simulink model "QCar2_Physical_02"  (R2024a)
settings: Solver=ode1  StartTime=0.0  StopTime=inf  FixedStep=Controller_Sample_Time  RelTol=1e-3  EnableMultiTasking=on
PreLoadFcn:
  | QCarSetup
values from neighbouring files (symbols this model uses):
  Audio_Sample_Time = 0.3    [QCarSetup.m]
  CSI_Sample_Time = 1/60    (= 0.0166666666667)    [QCarSetup.m]
  ImageDisplay_Sample_Time = 120*Controller_Sample_Time    (= 0.1)    [QCarSetup.m]
  LiDAR_Sample_Time = CSI_Sample_Time*3    (= 0.05)    [QCarSetup.m]
  NN_Sample_Time = RealSense_Sample_Time*1    (= 0.0333333333333)    [QCarSetup.m]
  RealSense_Sample_Time = CSI_Sample_Time*2    (= 0.0333333333333)    [QCarSetup.m]
undefined symbols (not defined in the file or in its folder): Cobra_Start, DiscIntNeverNeededParam, engine, gcbh, height, HIL, honk, Joystick_Sample_Time, JPEG, left, Point, put_me_down, qc_get_step_size, top, truck_start, video_display_show, width
libraries: quarc_library x53, simulink x4, simulink_extras x1, visiontextngfix x1
(part 1 of 2)
settings Model: SimulationMode=external  ExtModeTrigDuration=10000  Creator=PKaram  LastModifiedBy=admin
settings SolverCC: AlgebraicLoopSolver=TrustRegion  PositivePriorityOrder=on  AutoInsertRateTranBlk=on
settings DataIOCC: ReturnWorkspaceOutputs=off
settings OptimizationCC: ReuseModelBlockBuffer=off
settings DebuggingCC: ParameterPrecisionLossMsg=none  UnconnectedInputMsg=warning  UnconnectedOutputMsg=warning  UnconnectedLineMsg=warning  ArithmeticOperatorsInVariantConditions=warning
settings HardwareCC: ProdBitPerLong=64  ProdLargestAtomicInteger=LongLong  ProdLargestAtomicFloat=Double  ProdLongLongMode=on  ProdHWDeviceType=ARM Compatible->ARM 64-bit (LP64)
settings ModelReferenceCC: EnableRefExpFcnMdlSchedulingChecks=on
settings SFSimCC: SimUseLocalCustomCode=off  CustomCodeUndefinedFunction=UseInterfaceOnly
settings RTWCC: Description=QUARC Linux QCar2 Target Using Toolchain  SystemTargetFile=quarc_linux_qcar2.tlc  TemplateMakefile=quarc_linux_nvidia_tmf  RTWUseLocalCustomCode=off  Toolchain=QUARC linux_qcar2 | gmake (64-bit Windows)  BuildConfiguration=Faster Runs  GPUComputeCapability=3.5  DLArmComputeVersion=19.05
settings CodeAppCC: StateflowObjectComments=on
settings STFCustomTargetCC: ConcurrentExecutionCompliant=on  SystemTargetFile=quarc_linux_qcar2.tlc
settings GRTTargetCC: ParMdlRefBuildCompliant=off  CompOptLevelCompliant=off  CombineOutputUpdateFcns=off  MatFileLogging=off  CPPClassGenCompliant=off  GRTInterface=on  ExtMode=on  ExtModeMexFile=quarc_comm  ExtModeMexArgs='-w -d /tmp -uri %u', 'tcpip://192.168.2.11:17001'
settings ConfigComp: CovMetricSettings=dswe

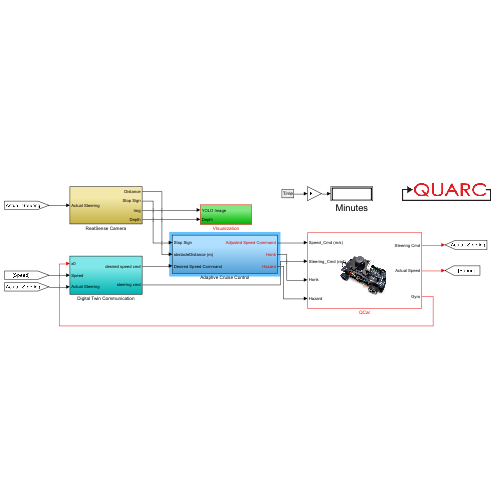
[thumbnail: Simulink's stored preview of the top-level diagram]
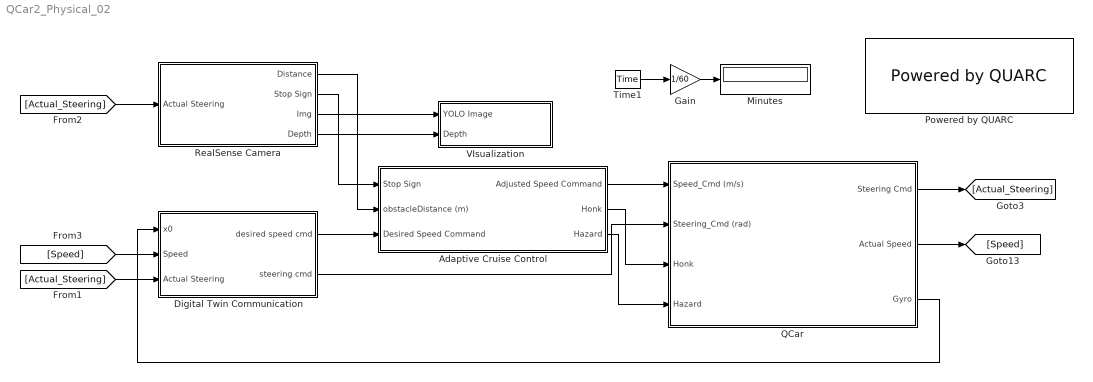
== system QCar2_Physical_02 ==
  Adaptive Cruise Control : Subsystem
  Digital Twin Communication : Subsystem
  Gain : Gain  Gain=1/60
  Minutes : Display
  Powered by QUARC : quarc_library/Logos/Powered by QUARC
  QCar : Subsystem
      mask Display: image('QCar.png'); % Use "Edit Image" on toolstrip to change.
  RealSense Camera : Subsystem
  Time1 : quarc_library/Sources/Time/Time  time_source=Wall clock  sample_time=qc_get_step_size
  VIsualization : Subsystem
  wires:
  QCar/1(Steering Cmd) -> [Actual_Steering]
  Time1/1 -> Gain/1
  Gain/1 -> Minutes/1
  RealSense Camera/1(Distance) -> Adaptive Cruise Control/2(obstacleDistance (m))
  Adaptive Cruise Control/1(Adjusted Speed Command) -> QCar/1(Speed_Cmd (m/s))
  Adaptive Cruise Control/2(Honk) -> QCar/3(Honk)
  QCar/2(Actual Speed) -> [Speed]
  [Actual_Steering] -> RealSense Camera/1(Actual Steering)
  RealSense Camera/2(Stop Sign) -> Adaptive Cruise Control/1(Stop Sign)
  Adaptive Cruise Control/3(Hazard) -> QCar/4(Hazard)
  QCar/3(Gyro) -> Digital Twin Communication/1(x0)
  [Speed] -> Digital Twin Communication/2(Speed)
  [Actual_Steering] -> Digital Twin Communication/3(Actual Steering)
  Digital Twin Communication/2(steering cmd) -> QCar/2(Steering_Cmd (rad))
  Digital Twin Communication/1(desired speed cmd) -> Adaptive Cruise Control/3(Desired Speed Command)
  RealSense Camera/3(Img) -> VIsualization/1(YOLO Image)
  RealSense Camera/4(Depth) -> VIsualization/2(Depth)

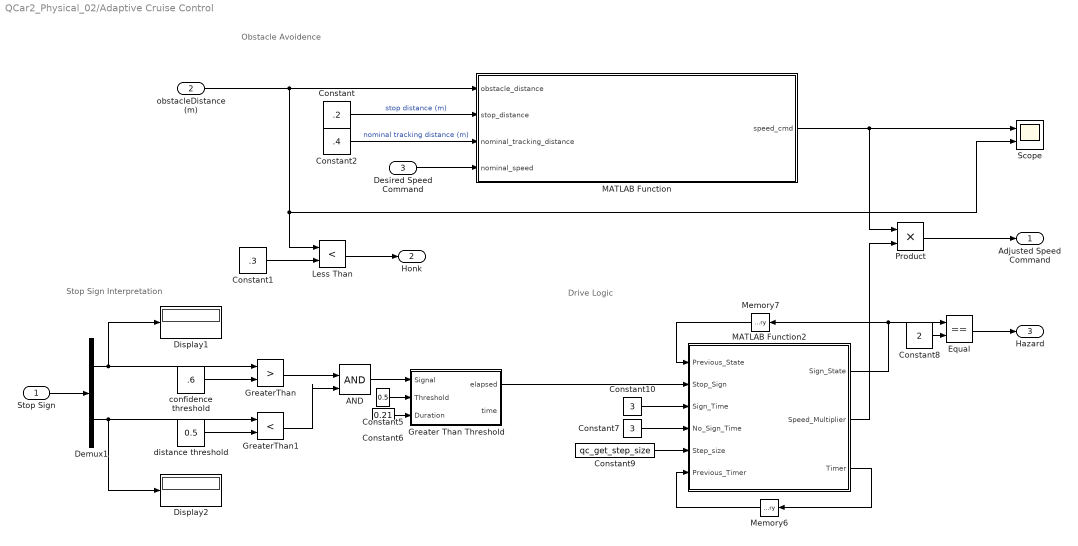
== system QCar2_Physical_02/Adaptive Cruise Control ==
  note: Drive Logic
  note: Obstacle Avoidence
  note: Stop Sign Interpretation
  Stop Sign : Inport
  obstacleDistance (m) : Inport  Port=2
  Desired Speed Command : Inport  Port=3
  AND : Logic  IconShape=distinctive  AllPortsSameDT=off
  Constant : Constant  Value=.2
  Constant1 : Constant  Value=.3
  Constant10 : Constant  Value=3
  Constant2 : Constant  Value=.4
  Constant5 : Constant  Value=0.5
  Constant6 : Constant  Value=0.21
  Constant7 : Constant  Value=3
  Constant8 : Constant  Value=2
  Constant9 : Constant  Value=qc_get_step_size
  Demux1 : Demux  Outputs=2
  Display1 : Display
  Display2 : Display
  Equal : RelationalOperator  Operator===  OutDataTypeStr=boolean  RndMeth=Simplest  InputSameDT=off
  Greater Than Threshold : Subsystem
  GreaterThan : RelationalOperator  Operator=>  OutDataTypeStr=boolean  RndMeth=Simplest  InputSameDT=off
  GreaterThan1 : RelationalOperator  Operator=<  OutDataTypeStr=boolean  RndMeth=Simplest  InputSameDT=off
  Less Than : RelationalOperator  Operator=<  OutDataTypeStr=boolean  RndMeth=Simplest  InputSameDT=off
  MATLAB Function : MATLAB Function  TreatAsAtomicUnit=on
  MATLAB Function2 : MATLAB Function  TreatAsAtomicUnit=on
  Memory6 : Memory  InheritSampleTime=on  LinearizeMemory=on  LinearizeAsDelay=on
  Memory7 : Memory  InitialCondition=1  InheritSampleTime=on  LinearizeMemory=on  LinearizeAsDelay=on
  Product : Product
  Scope : Scope  NumInputPorts=2
  confidence threshold : Constant  Value=.6
  distance threshold : Constant  Value=0.5
  Adjusted Speed Command : Outport  VectorParamsAs1DForOutWhenUnconnected=off
  Honk : Outport  Port=2
  Hazard : Outport  Port=3
  wires:
  Constant2/1 -> MATLAB Function/3(nominal_tracking_distance)  "nominal tracking distance (m)"
  Constant/1 -> MATLAB Function/2(stop_distance)  "stop distance (m)"
  obstacleDistance (m)/1 -> Less Than/1, Scope/2, MATLAB Function/1(obstacle_distance)
  Constant1/1 -> Less Than/2
  Less Than/1 -> Honk/1
  MATLAB Function/1(speed_cmd) -> Scope/1, Product/1
  Desired Speed Command/1 -> MATLAB Function/4(nominal_speed)
  Memory7/1 -> MATLAB Function2/1(Previous_State)
  Memory6/1 -> MATLAB Function2/6(Previous_Timer)
  MATLAB Function2/1(Sign_State) -> Equal/1, Memory7/1
  Constant9/1 -> MATLAB Function2/5(Step_size)
  Constant7/1 -> MATLAB Function2/4(No_Sign_Time)
  MATLAB Function2/2(Speed_Multiplier) -> Product/2
  Constant10/1 -> MATLAB Function2/3(Sign_Time)
  MATLAB Function2/3(Timer) -> Memory6/1
  Product/1 -> Adjusted Speed Command/1
  Stop Sign/1 -> Demux1/1
  Demux1/1 -> GreaterThan/1, Display1/1
  Demux1/2 -> Display2/1, GreaterThan1/1
  confidence threshold/1 -> GreaterThan/2
  distance threshold/1 -> GreaterThan1/2
  GreaterThan/1 -> AND/1
  GreaterThan1/1 -> AND/2
  AND/1 -> Greater Than Threshold/1(Signal)
  Constant5/1 -> Greater Than Threshold/2(Threshold)
  Constant6/1 -> Greater Than Threshold/3(Duration)
  Greater Than Threshold/1(elapsed) -> MATLAB Function2/2(Stop_Sign)
  Equal/1 -> Hazard/1
  Constant8/1 -> Equal/2

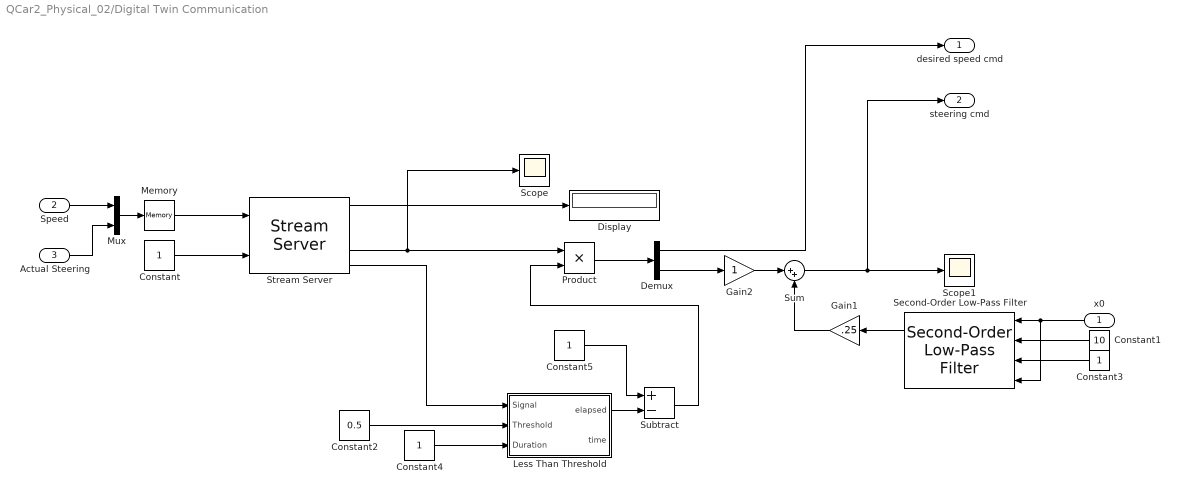
== system QCar2_Physical_02/Digital Twin Communication ==
  x0 : Inport
  Speed : Inport  Port=2
  Actual Steering : Inport  Port=3
  Constant{,3..5} (4 alike) : Constant
  Constant1 : Constant  Value=10
  Constant2 : Constant  Value=0.5
  Demux : Demux  Outputs=2
  Display : Display
  Gain1 : Gain  Gain=.25
  Gain2 : Gain
  Less Than Threshold : Subsystem
  Memory : Memory  InitialCondition=[0 0]
  Mux : Mux  Inputs=2
  Product : Product
  Scope : Scope
  Scope1 : Scope
  Second-Order Low-Pass Filter : quarc_library/Continuous/Second-Order Low-Pass Filter  params_source=External (input ports)  input_width=10  input_zeta=1  input_init=0
  Stream Server : quarc_library/Communications/Basic/Stream Server  uri_source=Specify via dialog (do not evaluate)  uri=tcpip://localhost:777  send_buffer_size=1460  receive_buffer_size=1460  byte_order=little endian (Intel - LSB first)  optimization=Minimum latency  send_options=Send most recent data  receive_options=Receive most recent data  default_value=[0 0]  sample_time=qc_get_step_size  active=off  implementation=Use blocking I/O in a separate thread  send_fifo_size=1000  receive_fifo_size=1000  send_priority=0  receive_priority=0  send_dimensions=off  receive_dimensions=off  max_dimensions=-1  data_type=Inherited via back propagation  type_expr=BusObject
      settings: AttributesFormatString="\"tcpip://localhost:777\""
  Subtract : Sum  Inputs=+-
  Sum : Sum  Inputs=|++
  desired speed cmd : Outport
  steering cmd : Outport  Port=2
  wires:
  Sum/1 -> steering cmd/1, Scope1/1
  Speed/1 -> Mux/1
  Constant1/1 -> Second-Order Low-Pass Filter/2
  Stream Server/1 -> Display/1
  x0/1 -> Second-Order Low-Pass Filter/4, Second-Order Low-Pass Filter/1
  Memory/1 -> Stream Server/1
  Demux/2 -> Gain2/1
  Gain1/1 -> Sum/2
  Less Than Threshold/1(elapsed) -> Subtract/2
  Constant2/1 -> Less Than Threshold/2(Threshold)
  Constant4/1 -> Less Than Threshold/3(Duration)
  Subtract/1 -> Product/2
  Stream Server/4 -> Scope/1, Product/1
  Actual Steering/1 -> Mux/2
  Constant3/1 -> Second-Order Low-Pass Filter/3
  Second-Order Low-Pass Filter/1 -> Gain1/1
  Mux/1 -> Memory/1
  Gain2/1 -> Sum/1
  Stream Server/5 -> Less Than Threshold/1(Signal)
  Constant5/1 -> Subtract/1
  Constant/1 -> Stream Server/2
  Product/1 -> Demux/1
  Demux/1 -> desired speed cmd/1

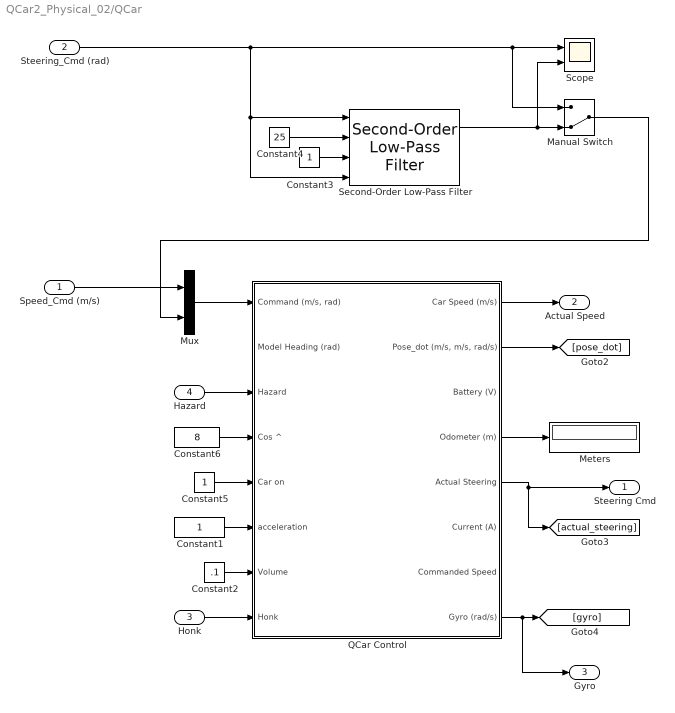
== system QCar2_Physical_02/QCar ==
  Speed_Cmd (m/s) : Inport
  Steering_Cmd (rad) : Inport  Port=2
  Honk : Inport  Port=3
  Hazard : Inport  Port=4
  Constant1 : Constant
  Constant2 : Constant  Value=.1
  Constant3 : Constant
  Constant4 : Constant  Value=25
  Constant5 : Constant
  Constant6 : Constant  Value=8
  Manual Switch : ManualSwitch  CurrentSetting=0
  Meters : Display
  Mux : Mux  Inputs=2
  QCar Control : Subsystem
  Scope : Scope  NumInputPorts=2
  Second-Order Low-Pass Filter : quarc_library/Continuous/Second-Order Low-Pass Filter  params_source=External (input ports)  input_width=1  input_zeta=1  input_init=0
  Steering Cmd : Outport
  Actual Speed : Outport  Port=2
  Gyro : Outport  Port=3
  wires:
  Mux/1 -> QCar Control/1("Command (m/s, rad)")
  Speed_Cmd (m/s)/1 -> Mux/1
  QCar Control/1(Car Speed (m/s)) -> Actual Speed/1
  QCar Control/2("Pose_dot (m/s, m/s, rad/s)") -> [pose_dot]
  QCar Control/5(Actual Steering) -> [actual_steering], Steering Cmd/1
  Constant6/1 -> QCar Control/4(Cos ^)
  Constant1/1 -> QCar Control/6(acceleration)
  Constant5/1 -> QCar Control/5(Car on)
  Constant2/1 -> QCar Control/7(Volume)
  Honk/1 -> QCar Control/8(Honk)
  QCar Control/4(Odometer (m)) -> Meters/1
  Hazard/1 -> QCar Control/3(Hazard)
  Manual Switch/1 -> Mux/2
  Second-Order Low-Pass Filter/1 -> Scope/2, Manual Switch/2
  Steering_Cmd (rad)/1 -> Manual Switch/1, Scope/1, Second-Order Low-Pass Filter/1, Second-Order Low-Pass Filter/4
  Constant3/1 -> Second-Order Low-Pass Filter/3
  Constant4/1 -> Second-Order Low-Pass Filter/2
  QCar Control/8(Gyro (rad/s)) -> Gyro/1, [gyro]

== system QCar2_Physical_02/RealSense Camera ==
  Actual Steering : Inport
  Constant8 : Constant  Value=50
  Constant9 : Constant
  Distance Comparison : Scope  Commented=on  NumInputPorts=3
  NN Classification : Scope
  Obstacle Detection : Subsystem
  Rate Transition : RateTransition
  Rate Transition2 : RateTransition
  Rate Transition4 : RateTransition
  RealSense Capture : Subsystem
  Second-Order Low-Pass Filter2 : quarc_library/Continuous/Second-Order Low-Pass Filter  params_source=External (input ports)  input_width=1  input_zeta=1  input_init=0
  Selector : Selector  NumberOfDimensions=2  InputPortWidth=3  IndexOptions=Index vector (dialog),Select all  Indices=2,1  OutputSizes=1,1
  Terminator : Terminator
  Transfer Fcn : TransferFcn  Numerator=[10]  Denominator=[1 10]
  Distance : Outport
  Stop Sign : Outport  Port=2
  Img : Outport  Port=3
  Depth : Outport  Port=4
  wires:
  Transfer Fcn/1 -> Rate Transition4/1
  Actual Steering/1 -> Transfer Fcn/1
  Constant9/1 -> Second-Order Low-Pass Filter2/3
  Rate Transition2/1 -> Second-Order Low-Pass Filter2/4, Second-Order Low-Pass Filter2/1
  Second-Order Low-Pass Filter2/2 -> Terminator/1
  RealSense Capture/2(New) -> Obstacle Detection/Enable
  Rate Transition4/1 -> Obstacle Detection/2(steering (rad))
  Constant8/1 -> Second-Order Low-Pass Filter2/2
  Second-Order Low-Pass Filter2/1 -> Distance/1, Distance Comparison/1
  RealSense Capture/4(Depth Aligned) -> Obstacle Detection/1(imageDepth)
  RealSense Capture/1(Classification Info) -> Rate Transition/1
  RealSense Capture/3(yolo image) -> Img/1
  Obstacle Detection/2(imageDepthForDisplay) -> Depth/1
  Selector/1 -> Stop Sign/1
  Rate Transition/1 -> NN Classification/1, Selector/1
  Obstacle Detection/1(distance (m)) -> Rate Transition2/1

== system QCar2_Physical_02/VIsualization ==
  YOLO Image : Inport
  Depth : Inport  Port=2
  Body Frame : quarc_library/Sinks/Figures/Polar Figure  figure_mode=Use figure window  figure_tag=figure1  axes_tag=axes1  plot_mode=Frame-based  minimum_rho=0  maximum_rho=4  minimum_theta=0  maximum_theta=360  zero_location=right  direction=clockwise  buffer_size=SPR  update_rate=1  sample_time=-1  initial_position="-1533.6667     -397.66667      638.66667      278.66667"  initial_visibility=off  line1_style=None  line1_width=0.5  line1_color=[0 0.4470 0.7410]  marker1=Point (.)  marker1_size=5  marker1_edge_color=[0 0.447059 0.741176]  marker1_face_color=[0 0.447059 0.741176]  line2_style=Solid line (-)  line2_width=0.5  line2_color=[0.85098 0.32549 0.0980392]  marker2=None  marker2_size=6  marker2_edge_color=[0.85098 0.32549 0.0980392]  marker2_face_color=[0.85098 0.32549 0.0980392]  line3_style=Solid line (-)  line3_width=0.5  line3_color=[0.929412 0.694118 0.12549]  marker3=None  marker3_size=6  marker3_edge_color=[0.929412 0.694118 0.12549]  marker3_face_color=[0.929412 0.694118 0.12549]  line4_style=Solid line (-)  line4_width=0.5  line4_color=[0.494118 0.184314 0.556863]  marker4=None  marker4_size=6  marker4_edge_color=[0.494118 0.184314 0.556863]  marker4_face_color=[0.494118 0.184314 0.556863]  line5_style=Solid line (-)  line5_width=0.5  line5_color=[0.466667 0.67451 0.188235]  marker5=None  marker5_size=6  marker5_edge_color=[0.466667 0.67451 0.188235]  marker5_face_color=[0.466667 0.67451 0.188235]
      settings: SourceProductName=QUARC Targets
  LiDAR : Subsystem
  Newer Depth : Subsystem  LoadFcn=set_param(gcbh, 'UserData', gcb);  StartFcn=video_display_show([gcb, '/Video Display'], 'add', gcb);  mask(Video Compressed Display){algorithm=JPEG, quality=50, sample_time=-1, use_hardware=on}
      mask prompts: algorithm "Compression algorithm:"; quality "Compression quality (0-100):"; sample_time "Sample time (seconds):"; use_hardware "Use hardware acceleration for video display"
      mask help: Displays a video stream on the host, using compression to minimize bandwidth.
      mask init:
      | qc_set_display('Video\nCompressed\nDisplay');
      settings: UndoDeleteFcn=set_param(gcbh, 'UserData', gcb);  OpenFcn=video_display_show([gcb, '/Video Display'], 'show', gcb);  PreDeleteFcn=video_display_show([gcb, '/Video Display'], 'delete');
      settings: CopyFcn=|
      | set_param(gcbh, 'UserData', gcb);
      | set_param(gcbh, 'LinkStatus', 'none');
      settings: NameChangeFcn=|
      | video_display_show([get_param(gcbh, 'UserData'), '/Video Display'], 'rename', [gcb, '/Video Display']);
      | video_display_show([gcb, '/Video Display'], 'add', gcb);
      | set_param(gcbh, 'UserData', gcb);
      mask Help: web(qc_get_block_help_path(gcb));
      mask TypeOptions algorithm: Image Compress/algorithm
      mask TypeOptions quality: Image Compress/quality
      mask TypeOptions sample_time: Video Display/sample_time
      mask TypeOptions use_hardware: Video Display/use_hardware
      mask Display:
      | patch([0.98591 0.98591 0.62618 0.59072 0.56147   0.536   0.536  0.5441 0.56912 0.59207 0.60881 0.62276 0.63527 0.64364  0.6485  0.6485 0.64706 0.64499 0.63662 0.62411 0.61232 0.59837 0.58307 0.56147   0.536   0.536  0.5441  0.5747 0.60953 0.63662 0.67001  0.7034 0.72851 0.75425 0.77927 0.80294 0.82454 0.84119 0.85865 0.87395 0.88574 0.89339  0.8969 0.89969 0.89969 0.89267  0.8816 0.87044 0.85649  0.8384 0.81824 0.80294 0.78764 0.77513 0.76676 0.75776 0.76397 0.77513 0.79178 0.80987 0.82796 0.84326 0.86207 0.98528],[0.18689 0.05522 0.05522 0.05171 0.05171    0.05 0.18338 0.18338 0.19148 0.20435 0.22298 0.24863 0.28589 0.33125 0.38138 0.55139 0.59801 0.63761 0.68189 0.72149 0.74939 0.76694 0.77855 0.79367 0.79952 0.92768 0.92768 0.92768 0.92417 0.92066 0.91364  0.9032 0.89384 0.88106 0.86594 0.85073 0.82634 0.80537 0.77855 0.74363 0.70403 0.65858 0.61079 0.59099 0.41513 0.37202 0.31847 0.29048 0.25556 0.23342  0.2102 0.19382 0.18221 0.17285 0.16943 0.16124  0.1589 0.16241 0.16709 0.17168  0.1787 0.18221 0.18689 0.18689],[0.9,0.90,0.91])
      | patch([0.536 0.52601 0.46823 0.44528 0.41603 0.39101 0.35555 0.33116 0.31451 0.29291  0.2804 0.26717 0.25322 0.23999 0.22406 0.20732 0.19337 0.17528 0.15935 0.14396 0.13217 0.11759 0.10922 0.10085 0.09671 0.09392 0.09041 0.08906 0.08906 0.09464  0.0995 0.10778 0.11894 0.13145 0.14675 0.16349 0.17672 0.19409 0.20732 0.22406 0.23999 0.26159 0.27833 0.29849 0.31793 0.33602 0.35411 0.37085 0.39245 0.41603   0.536   0.536 0.53159 0.46409   0.446 0.42026 0.39587 0.37571 0.36113 0.34925 0.34088 0.33809 0.33809 0.34088 0.34583 0.35627 0.36392 0.38129 0.39587 0.41117 0.42719 0.44672  0.4676 0.48353 0.48353 0.52394   0.536],[0.05 0.04829 0.04712 0.04712 0.04829 0.05063 0.05405 0.05873 0.06107 0.06692 0.07043 0.07619 0.08087 0.08672 0.09482 0.10652 0.11696 0.13325  0.1508 0.17168 0.19499 0.22415 0.25439 0.28472 0.31379 0.35456 0.38489 0.41513 0.58055 0.63878 0.68774 0.72149 0.75641 0.78089 0.80537 0.82859 0.84029 0.85658 0.86594 0.87404  0.8834 0.89267 0.90086 0.90788 0.91247 0.91832 0.92066   0.923 0.92651 0.92768 0.92768 0.79952 0.79952 0.79952 0.79718 0.78899 0.77153 0.75056 0.72149 0.68072 0.62249  0.5549 0.41396 0.37085 0.33242 0.28121 0.25205 0.22181 0.20552 0.19499 0.18572 0.18221 0.17753 0.17636 0.17753  0.1787  0.1787],[0.9,0.90,0.91])
      | disp('Video\nCompressed\nDisplay');
  Rate Timing Plots : Subsystem
  Speed_Tracking : Scope  NumInputPorts=2
  Yolo Image : Subsystem  LoadFcn=set_param(gcbh, 'UserData', gcb);  StartFcn=video_display_show([gcb, '/Video Display'], 'add', gcb);  mask(Video Compressed Display){algorithm=JPEG, quality=50, sample_time=-1, use_hardware=on}
      mask prompts: algorithm "Compression algorithm:"; quality "Compression quality (0-100):"; sample_time "Sample time (seconds):"; use_hardware "Use hardware acceleration for video display"
      mask help: Displays a video stream on the host, using compression to minimize bandwidth.
      mask init:
      | qc_set_display('Video\nCompressed\nDisplay');
      settings: UndoDeleteFcn=set_param(gcbh, 'UserData', gcb);  OpenFcn=video_display_show([gcb, '/Video Display'], 'show', gcb);  PreDeleteFcn=video_display_show([gcb, '/Video Display'], 'delete');
      settings: CopyFcn=|
      | set_param(gcbh, 'UserData', gcb);
      | set_param(gcbh, 'LinkStatus', 'none');
      settings: NameChangeFcn=|
      | video_display_show([get_param(gcbh, 'UserData'), '/Video Display'], 'rename', [gcb, '/Video Display']);
      | video_display_show([gcb, '/Video Display'], 'add', gcb);
      | set_param(gcbh, 'UserData', gcb);
      mask Help: web(qc_get_block_help_path(gcb));
      mask TypeOptions algorithm: Image Compress/algorithm
      mask TypeOptions quality: Image Compress/quality
      mask TypeOptions sample_time: Video Display/sample_time
      mask TypeOptions use_hardware: Video Display/use_hardware
      mask Display:
      | patch([0.98591 0.98591 0.62618 0.59072 0.56147   0.536   0.536  0.5441 0.56912 0.59207 0.60881 0.62276 0.63527 0.64364  0.6485  0.6485 0.64706 0.64499 0.63662 0.62411 0.61232 0.59837 0.58307 0.56147   0.536   0.536  0.5441  0.5747 0.60953 0.63662 0.67001  0.7034 0.72851 0.75425 0.77927 0.80294 0.82454 0.84119 0.85865 0.87395 0.88574 0.89339  0.8969 0.89969 0.89969 0.89267  0.8816 0.87044 0.85649  0.8384 0.81824 0.80294 0.78764 0.77513 0.76676 0.75776 0.76397 0.77513 0.79178 0.80987 0.82796 0.84326 0.86207 0.98528],[0.18689 0.05522 0.05522 0.05171 0.05171    0.05 0.18338 0.18338 0.19148 0.20435 0.22298 0.24863 0.28589 0.33125 0.38138 0.55139 0.59801 0.63761 0.68189 0.72149 0.74939 0.76694 0.77855 0.79367 0.79952 0.92768 0.92768 0.92768 0.92417 0.92066 0.91364  0.9032 0.89384 0.88106 0.86594 0.85073 0.82634 0.80537 0.77855 0.74363 0.70403 0.65858 0.61079 0.59099 0.41513 0.37202 0.31847 0.29048 0.25556 0.23342  0.2102 0.19382 0.18221 0.17285 0.16943 0.16124  0.1589 0.16241 0.16709 0.17168  0.1787 0.18221 0.18689 0.18689],[0.9,0.90,0.91])
      | patch([0.536 0.52601 0.46823 0.44528 0.41603 0.39101 0.35555 0.33116 0.31451 0.29291  0.2804 0.26717 0.25322 0.23999 0.22406 0.20732 0.19337 0.17528 0.15935 0.14396 0.13217 0.11759 0.10922 0.10085 0.09671 0.09392 0.09041 0.08906 0.08906 0.09464  0.0995 0.10778 0.11894 0.13145 0.14675 0.16349 0.17672 0.19409 0.20732 0.22406 0.23999 0.26159 0.27833 0.29849 0.31793 0.33602 0.35411 0.37085 0.39245 0.41603   0.536   0.536 0.53159 0.46409   0.446 0.42026 0.39587 0.37571 0.36113 0.34925 0.34088 0.33809 0.33809 0.34088 0.34583 0.35627 0.36392 0.38129 0.39587 0.41117 0.42719 0.44672  0.4676 0.48353 0.48353 0.52394   0.536],[0.05 0.04829 0.04712 0.04712 0.04829 0.05063 0.05405 0.05873 0.06107 0.06692 0.07043 0.07619 0.08087 0.08672 0.09482 0.10652 0.11696 0.13325  0.1508 0.17168 0.19499 0.22415 0.25439 0.28472 0.31379 0.35456 0.38489 0.41513 0.58055 0.63878 0.68774 0.72149 0.75641 0.78089 0.80537 0.82859 0.84029 0.85658 0.86594 0.87404  0.8834 0.89267 0.90086 0.90788 0.91247 0.91832 0.92066   0.923 0.92651 0.92768 0.92768 0.79952 0.79952 0.79952 0.79718 0.78899 0.77153 0.75056 0.72149 0.68072 0.62249  0.5549 0.41396 0.37085 0.33242 0.28121 0.25205 0.22181 0.20552 0.19499 0.18572 0.18221 0.17753 0.17636 0.17753  0.1787  0.1787],[0.9,0.90,0.91])
      | disp('Video\nCompressed\nDisplay');
  wires:
  YOLO Image/1 -> Yolo Image/1(In1)
  LiDAR/1(Distance) -> Body Frame/1
  LiDAR/2(Heading) -> Body Frame/2
  Depth/1 -> Newer Depth/1(In1)
  [desiredSpd] -> Speed_Tracking/1
  [measuredSpd] -> Speed_Tracking/2

== system QCar2_Physical_02/Adaptive Cruise Control/Greater Than Threshold ==
  Signal : Inport
  Threshold : Inport  Port=2
  Duration : Inport  Port=3
  Data Type Conversion : DataTypeConversion  SaturateOnIntegerOverflow=off  RndMeth=Floor
  Discrete-Time Integrator : DiscreteIntegrator  Priority=1  ExternalReset=level  SampleTime=qc_get_step_size  ICPrevOutput=DiscIntNeverNeededParam  ICPrevScaledInput=DiscIntNeverNeededParam
  Logical Operator : Logic  Operator=NOT  AllPortsSameDT=off  OutDataTypeStr=boolean
  Relational Operator : RelationalOperator  InputSameDT=off
  Relational Operator1 : RelationalOperator  InputSameDT=off
  elapsed : Outport  VectorParamsAs1DForOutWhenUnconnected=off
  time : Outport  Port=2  VectorParamsAs1DForOutWhenUnconnected=off
  wires:
  Data Type Conversion/1 -> Discrete-Time Integrator/1
  Signal/1 -> Relational Operator/1
  Threshold/1 -> Relational Operator/2
  Relational Operator/1 -> Data Type Conversion/1, Logical Operator/1
  Logical Operator/1 -> Discrete-Time Integrator/2
  Discrete-Time Integrator/1 -> Relational Operator1/1, time/1
  Duration/1 -> Relational Operator1/2
  Relational Operator1/1 -> elapsed/1

== system QCar2_Physical_02/Digital Twin Communication/Less Than Threshold ==
  Signal : Inport
  Threshold : Inport  Port=2
  Duration : Inport  Port=3
  Data Type Conversion : DataTypeConversion  SaturateOnIntegerOverflow=off  RndMeth=Floor
  Discrete-Time Integrator : DiscreteIntegrator  Priority=1  ExternalReset=level  SampleTime=qc_get_step_size  ICPrevOutput=DiscIntNeverNeededParam  ICPrevScaledInput=DiscIntNeverNeededParam
  Logical Operator : Logic  Operator=NOT  AllPortsSameDT=off  OutDataTypeStr=boolean
  Relational Operator : RelationalOperator  Operator=<  InputSameDT=off
  Relational Operator1 : RelationalOperator  InputSameDT=off
  elapsed : Outport  VectorParamsAs1DForOutWhenUnconnected=off
  time : Outport  Port=2  VectorParamsAs1DForOutWhenUnconnected=off
  wires:
  Relational Operator1/1 -> elapsed/1
  Duration/1 -> Relational Operator1/2
  Discrete-Time Integrator/1 -> time/1, Relational Operator1/1
  Logical Operator/1 -> Discrete-Time Integrator/2
  Relational Operator/1 -> Logical Operator/1, Data Type Conversion/1
  Threshold/1 -> Relational Operator/2
  Signal/1 -> Relational Operator/1
  Data Type Conversion/1 -> Discrete-Time Integrator/1

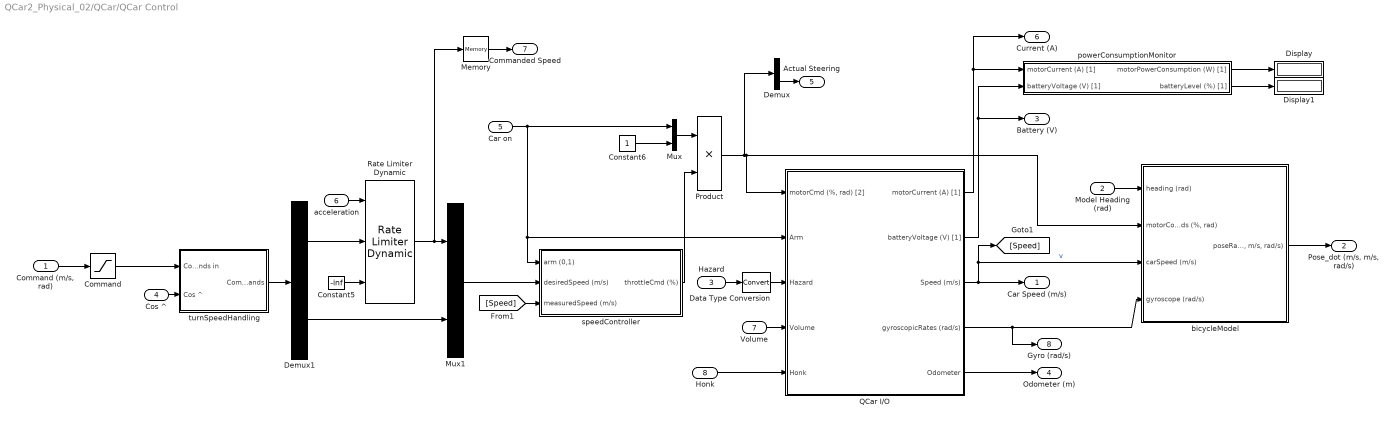
== system QCar2_Physical_02/QCar/QCar Control ==
  "Command (m/s, rad)" : Inport
  Model Heading (rad) : Inport  Port=2
  Hazard : Inport  Port=3
  Cos ^ : Inport  Port=4
  Car on : Inport  Port=5
  acceleration : Inport  Port=6
  Volume : Inport  Port=7
  Honk : Inport  Port=8
  Command : Saturate  UpperLimit=[3 .6]  LowerLimit=-[3 .6]
  Constant5 : Constant  Value=-inf
  Constant6 : Constant
  Data Type Conversion : DataTypeConversion  SaturateOnIntegerOverflow=off  RndMeth=Floor
  Demux : Demux  Outputs=2
  Demux1 : Demux  Outputs=2
  Display : Display
      settings: Decimation=100
  Display1 : Display
      settings: Decimation=100
  Memory : Memory
  Mux : Mux  Inputs=2
  Mux1 : Mux  Inputs=2
  Product : Product
  QCar I/O : Subsystem
  Rate Limiter Dynamic : simulink/Discontinuities/Rate Limiter Dynamic
  bicycleModel : Subsystem
  powerConsumptionMonitor : Subsystem
  speedController : Subsystem
  turnSpeedHandling : Subsystem
  Car Speed (m/s) : Outport
  "Pose_dot (m/s, m/s, rad/s)" : Outport  Port=2
  Battery (V) : Outport  Port=3
  Odometer (m) : Outport  Port=4
  Actual Steering : Outport  Port=5
  Current (A) : Outport  Port=6
  Commanded Speed : Outport  Port=7
  Gyro (rad/s) : Outport  Port=8
  wires:
  QCar I/O/2(batteryVoltage (V) [1]) -> Battery (V)/1, powerConsumptionMonitor/2(batteryVoltage (V) [1])
  powerConsumptionMonitor/1(motorPowerConsumption (W) [1]) -> Display/1
  QCar I/O/1(motorCurrent (A) [1]) -> Current (A)/1, powerConsumptionMonitor/1(motorCurrent (A) [1])
  Model Heading (rad)/1 -> bicycleModel/1(heading (rad))
  powerConsumptionMonitor/2(batteryLevel (%) [1]) -> Display1/1
  QCar I/O/4(gyroscopicRates (rad/s)) -> Gyro (rad/s)/1, bicycleModel/4(gyroscope (rad/s))
  bicycleModel/1("poseRate (m/s, m/s, rad/s)") -> "Pose_dot (m/s, m/s, rad/s)"/1
  Product/1 -> QCar I/O/1("motorCmd (%, rad) [2]"), bicycleModel/2("motorCommands (%, rad)"), Demux/1
  Car on/1 -> QCar I/O/2(Arm), speedController/1(arm (0,1)), Mux/1
  QCar I/O/5(Odometer) -> Odometer (m)/1
  [Speed] -> speedController/3(measuredSpeed (m/s))
  Demux/2 -> Actual Steering/1
  Hazard/1 -> Data Type Conversion/1
  Cos ^/1 -> turnSpeedHandling/2(Cos ^)
  Data Type Conversion/1 -> QCar I/O/3(Hazard)
  speedController/1(throttleCmd (%)) -> Product/2
  Mux/1 -> Product/1
  Constant6/1 -> Mux/2
  Volume/1 -> QCar I/O/4(Volume)
  QCar I/O/3(Speed (m/s)) -> [Speed], bicycleModel/3(carSpeed (m/s)), Car Speed (m/s)/1  "v"
  "Command (m/s, rad)"/1 -> Command/1
  Demux1/1 -> Rate Limiter Dynamic/2
  Rate Limiter Dynamic/1 -> Memory/1, Mux1/1
  Constant5/1 -> Rate Limiter Dynamic/3
  acceleration/1 -> Rate Limiter Dynamic/1
  Demux1/2 -> Mux1/2
  turnSpeedHandling/1(Commands) -> Demux1/1
  Mux1/1 -> speedController/2(desiredSpeed (m/s))
  Command/1 -> turnSpeedHandling/1(Commands in)
  Honk/1 -> QCar I/O/5(Honk)
  Memory/1 -> Commanded Speed/1

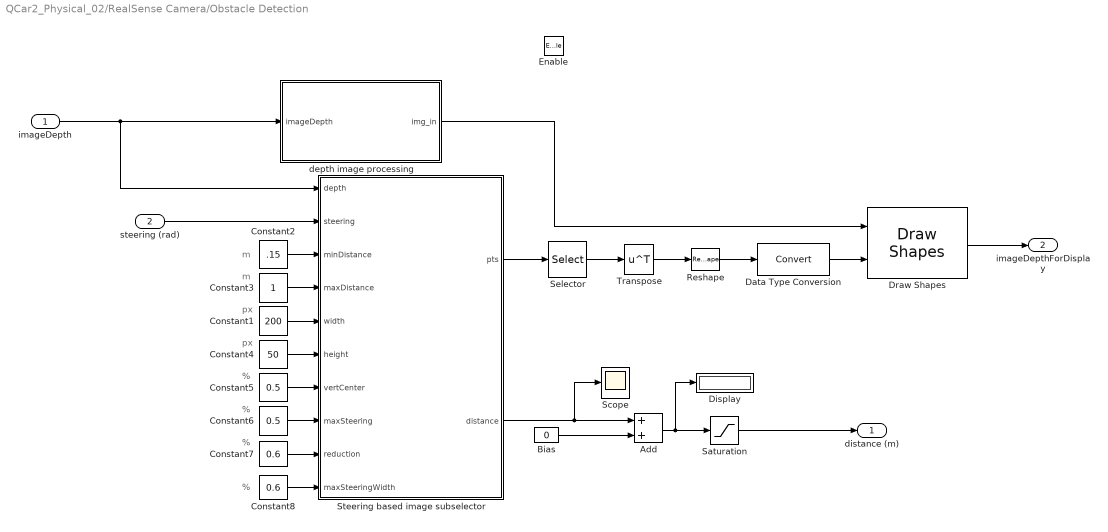
== system QCar2_Physical_02/RealSense Camera/Obstacle Detection ==
  note: %
  note: m
  note: m
  note: %
  note: px
  note: px
  note: %
  note: %
  imageDepth : Inport
  steering (rad) : Inport  Port=2
  Enable : EnablePort  PropagateVarSize=During execution
  Add : Sum
  Bias : Constant  Value=0
  Constant1 : Constant  Value=200
  Constant2 : Constant  Value=.15
  Constant3 : Constant
  Constant4 : Constant  Value=50
  Constant5 : Constant  Value=0.5
  Constant6 : Constant  Value=0.5
  Constant7 : Constant  Value=0.6
  Constant8 : Constant  Value=0.6
  Data Type Conversion : DataTypeConversion  SaturateOnIntegerOverflow=off  RndMeth=Floor
  Display : Display
  Draw Shapes : visiontextngfix/Draw Shapes  shape=Polygons  fill=off  lineWidth=1  fillClrSource=Specify via dialog  display=White  intensity=200  color=[200 255 100]  opacity=0.6  viewport=Entire image  antialiasing=off  inType=Obsolete  imagePorts=One multidimensional signal  roundingMode=Floor  overflowMode=off  memoryMode=Specify word length  memoryWordLength=16  prodOutputMode=Binary point scaling  prodOutputWordLength=32  prodOutputFracLength=14  memoryFracLength=15
  Reshape : Reshape  OutputDimensionality=Customize  OutputDimensions=[1,8]
  Saturation : Saturate  UpperLimit=2  LowerLimit=0.05
  Scope : Scope
  Selector : Selector  NumberOfDimensions=2  InputPortWidth=2  IndexOptions=Index vector (dialog),Index vector (dialog)  Indices=[1 2 3 4],[2 1]  OutputSizes=1,1
  Steering based image subselector : MATLAB Function  TreatAsAtomicUnit=on
  Transpose : Math  Operator=transpose
  depth image processing : Subsystem
  distance (m) : Outport  VectorParamsAs1DForOutWhenUnconnected=off
  imageDepthForDisplay : Outport  Port=2  VectorParamsAs1DForOutWhenUnconnected=off
  wires:
  Constant6/1 -> Steering based image subselector/8(maxSteering)
  Steering based image subselector/2(distance) -> Add/1, Scope/1
  Constant5/1 -> Steering based image subselector/7(vertCenter)
  Constant4/1 -> Steering based image subselector/6(height)
  Constant1/1 -> Steering based image subselector/5(width)
  Constant3/1 -> Steering based image subselector/4(maxDistance)
  Constant2/1 -> Steering based image subselector/3(minDistance)
  steering (rad)/1 -> Steering based image subselector/2(steering)
  Steering based image subselector/1(pts) -> Selector/1
  Bias/1 -> Add/2
  Add/1 -> Saturation/1, Display/1
  Saturation/1 -> distance (m)/1
  Constant7/1 -> Steering based image subselector/9(reduction)
  Constant8/1 -> Steering based image subselector/10(maxSteeringWidth)
  depth image processing/1(img_in) -> Draw Shapes/1
  imageDepth/1 -> Steering based image subselector/1(depth), depth image processing/1(imageDepth)
  Reshape/1 -> Data Type Conversion/1
  Draw Shapes/1 -> imageDepthForDisplay/1
  Data Type Conversion/1 -> Draw Shapes/2
  Selector/1 -> Transpose/1
  Transpose/1 -> Reshape/1

== system QCar2_Physical_02/RealSense Camera/RealSense Capture ==
  note: depth filter
  Depth Image : quarc_library/Multimedia/Video3D Capture  object_name=RealSense  stream_type=Depth  stream_index=0  resolution=640 x 480  width=640  height=480  output_format=Distance in meters (HxW)  data_type=single  sample_time=RealSense_Sample_Time  camera_intrinsics=on  depth_scale=on  brightness_override=Do not override  brightness=50.0  contrast_override=Do not override  contrast=50.0  hue_override=Do not override  hue=50.0  saturation_override=Do not override  saturation=50.0  sharpness_override=Do not override  sharpness=50.0  gamma_override=Do not override  gamma=50.0  gain_override=Do not override  gain=50.0  backlightcompensation_override=Do not override  backlightcompensation=50.0  whitebalance_override=Automatic white balance  whitebalance=50.0  exposure_override=Automatic exposure  exposure=30.0  emitter=Enable laser emitter  preset=Do not set camera presets
  Image Align : quarc_library/Image Processing/Generic/Image Align  direction=Depth to other
      settings: SourceProductName=QUARC Targets
  RGB Images : quarc_library/Multimedia/Video3D Capture  object_name=RealSense  stream_type=RGB  stream_index=0  resolution=640 x 480  width=640  height=480  output_format=MATLAB RGB (HxWx3)  data_type=uint8  sample_time=RealSense_Sample_Time*1  camera_intrinsics=on  depth_scale=off  brightness_override=Do not override  brightness=50.0  contrast_override=Do not override  contrast=50.0  hue_override=Do not override  hue=50.0  saturation_override=Do not override  saturation=50.0  sharpness_override=Do not override  sharpness=50.0  gamma_override=Do not override  gamma=50.0  gain_override=Do not override  gain=50.0  backlightcompensation_override=Do not override  backlightcompensation=50.0  whitebalance_override=Automatic white balance  whitebalance=50.0  exposure_override=Automatic exposure  exposure=30.0  emitter=Enable laser emitter  preset=Do not set camera presets
  Scope : Scope
  Subsystem : Subsystem
  Terminator{,1..4} (5 alike) : Terminator
  Video3D Extrinsics : quarc_library/Multimedia/Video3D Extrinsics  object_name=RealSense  from_block=RealSense Camera/RealSense Capture/Depth Image  to_block=RealSense Camera/RealSense Capture/RGB Images  sample_time=qc_get_step_size * ceil(1/30 / qc_get_step_size)
      settings: SourceProductName=QUARC Targets
  Video3D Initialize : quarc_library/Multimedia/Video3D Initialize  object_name=RealSense  source=Device  identifier=0  file=sample.bag  sample_time=RealSense_Sample_Time  active=on
  yolo_stream : Subsystem
  Classification Info : Outport
  New : Outport  Port=2
  yolo image : Outport  Port=3
  Depth Aligned : Outport  Port=4
  wires:
  Depth Image/4 -> New/1
  Depth Image/2 -> Terminator4/1
  Depth Image/3 -> Terminator3/1
  Video3D Initialize/1 -> Terminator/1
  RGB Images/1 -> Image Align/4, yolo_stream/2(rgb)  "rgb"
  RGB Images/2 -> Terminator1/1
  RGB Images/3 -> Terminator2/1
  RGB Images/4 -> Scope/1, yolo_stream/3(new)  "rgb new"
  Depth Image/5 -> Image Align/2
  Depth Image/8 -> Image Align/3
  RGB Images/5 -> Image Align/5
  Video3D Extrinsics/1 -> Image Align/6
  Image Align/1 -> yolo_stream/1(depth), Depth Aligned/1  "depth"
  yolo_stream/2(Classification info) -> Classification Info/1
  yolo_stream/1(Annotated Image) -> yolo image/1
  Depth Image/1 -> Subsystem/1(In1)
  Subsystem/1(Out1) -> Image Align/1

== system QCar2_Physical_02/VIsualization/LiDAR ==
  Bias : Bias  Bias=-pi/2+1*1.5*pi/180  SaturateOnIntegerOverflow=off
  Scope : Scope
  captureLIDAR : Subsystem
  Distance : Outport
  Heading : Outport  Port=2
  wires:
  captureLIDAR/1(distances (m)) -> Distance/1
  captureLIDAR/2(Heading (rad)) -> Bias/1
  Bias/1 -> Heading/1
  captureLIDAR/4(new) -> Scope/1

== system QCar2_Physical_02/VIsualization/Newer Depth ==
  In1 : Inport
  Channel : quarc_library/Signal Routing/Channel  channel=0  buffer_size=1
  Image Compress : quarc_library/Image Processing/Generic/Image Compress  algorithm=JPEG  source=Internal dialog parameter  quality=quality  output_dim=-1
  Video Display : quarc_library/Multimedia/Video Display  Tag=QCar2_Physical_02/VIsualization/Newer Depth/Video Display  sample_time=sample_time  use_hardware=on
  wires:
  Image Compress/1 -> Channel/1
  In1/1 -> Image Compress/1
  Channel/1 -> Video Display/1

== system QCar2_Physical_02/VIsualization/Rate Timing Plots ==
  Audio : Scope
  CSI : Scope
  Control : Scope
  Image Displays : Scope
  Joystick : Scope  Commented=on
  LCD : Scope
  LiDAR : Scope
  NN Rate : Scope
  RealSense : Scope
  monitorTiming : Subsystem
  monitorTiming1 : Subsystem
  monitorTiming2 : Subsystem
  monitorTiming3 : Subsystem
  monitorTiming4 : Subsystem  Commented=on
  monitorTiming5 : Subsystem
  monitorTiming6 : Subsystem
  monitorTiming7 : Subsystem
  monitorTiming8 : Subsystem
  wires:
  monitorTiming/1(Timing (s)) -> CSI/1
  monitorTiming1/1(Timing (s)) -> Control/1
  monitorTiming3/1(Timing (s)) -> Image Displays/1
  monitorTiming4/1(Timing (s)) -> Joystick/1
  monitorTiming2/1(Timing (s)) -> RealSense/1
  monitorTiming5/1(Timing (s)) -> LiDAR/1
  monitorTiming6/1(Timing (s)) -> NN Rate/1
  monitorTiming7/1(Timing (s)) -> LCD/1
  monitorTiming8/1(Timing (s)) -> Audio/1

== system QCar2_Physical_02/VIsualization/Yolo Image ==
  In1 : Inport
  Channel : quarc_library/Signal Routing/Channel  channel=1  buffer_size=1
  Image Compress : quarc_library/Image Processing/Generic/Image Compress  algorithm=JPEG  source=Internal dialog parameter  quality=quality  output_dim=-1
  Video Display : quarc_library/Multimedia/Video Display  Tag=QCar2_Physical_02/VIsualization/Yolo Image/Video Display  sample_time=sample_time  use_hardware=on
  wires:
  Image Compress/1 -> Channel/1
  In1/1 -> Image Compress/1
  Channel/1 -> Video Display/1

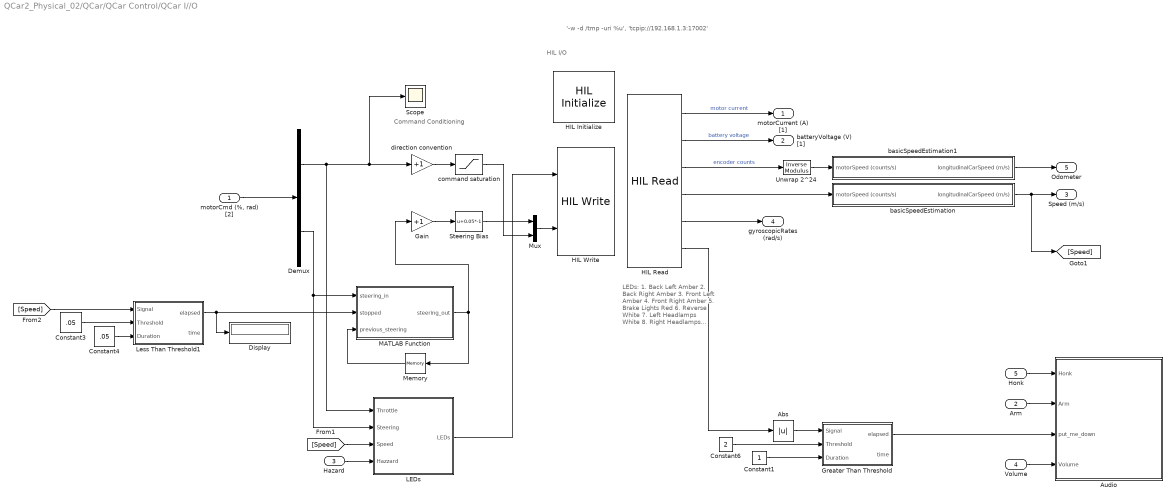
== system QCar2_Physical_02/QCar/QCar Control/QCar I//O ==
  note: '-w -d /tmp -uri %u', 'tcpip://192.168.1.3:17002'
  note: Command Conditioning
  note: HIL I/O
  note: LEDs:
      | 1. Back Left Amber
      | 2. Back Right Amber
      | 3. Front Left Amber
      | 4. Front Right Amber
      | 5. Brake Lights Red
      | 6. Reverse White
      | 7. Left Headlamps White
      | 8. Right Headlamps White
  "motorCmd (%, rad) [2]" : Inport
  Arm : Inport  Port=2
  Hazard : Inport  Port=3
  Volume : Inport  Port=4
  Honk : Inport  Port=5
  Abs : Abs  SaturateOnIntegerOverflow=off
  Audio : Subsystem
  Constant1 : Constant
  Constant3 : Constant  Value=.05
  Constant4 : Constant  Value=.05
  Constant6 : Constant  Value=2
  Demux : Demux  Outputs=2
  Display : Display
  Gain : Gain  Gain=+1
  Greater Than Threshold : Subsystem
  HIL Initialize : quarc_library/Data Acquisition/Generic/Configuration/HIL Initialize  object_name=HIL-1  board_type=qcar2  board_number=0  board_options=gyro_fs=250;gyro_rate=500;gyro_bw=125;gyro_ord=3;accel_fs=16;accel_rate=1000;accel_bw=250;accel_ord=3;temp_bw=4000;enc0_dir=0;enc1_dir=0;enc2_dir=0;steer_bias=0.05;  exclusive=off  active=on  hardware_clocks=[]  clock_modes=[]  initial_clock_frequencies=[]  set_clock_params_at_start=off  set_clock_params_at_switch_in=off  set_clock_frequencies_at_start=off  set_clock_frequencies_at_switch_in=off  analog_input_channels=[0:4]  analog_input_configurations=[]  analog_input_maximums=[3.3]  analog_input_minimums=[0]  set_analog_input_params_at_start=off  set_analog_input_params_at_switch_in=off  analog_output_channels=[]  analog_output_maximums=[]  analog_output_minimums=[]  initial_analog_outputs=[]  final_analog_outputs=[]  watchdog_analog_outputs=[]  set_analog_output_params_at_start=off  set_analog_output_params_at_switch_in=off  set_analog_outputs_at_start=off  set_analog_outputs_at_switch_in=off  set_analog_outputs_at_terminate=off  set_analog_outputs_at_switch_out=off  set_analog_outputs_on_watchdog=off  digital_input_channels=[0:14]  digital_output_channels=[11:26]  digital_output_configuration=[]  initial_digital_outputs=[0]  final_digital_outputs=[0]  watchdog_digital_outputs=[0]  set_digital_output_params_at_start=off  set_digital_output_params_at_switch_in=off  set_digital_outputs_at_start=on  set_digital_outputs_at_switch_in=off  set_digital_outputs_at_terminate=on  set_digital_outputs_at_switch_out=off  set_digital_outputs_on_watchdog=off  encoder_channels=[0:2]  quadrature=[4]  encoder_filter_frequency=100e6/1  initial_encoder_counts=[0]  set_encoder_params_at_start=on  set_encoder_params_at_switch_in=off  set_encoder_counts_at_start=on  set_encoder_counts_at_switch_in=off  pwm_channels=[0:1]  pwm_modes=[0]  pwm_frequency=180e6/4096  pwm_configuration=[0]  pwm_alignment=[0]  pwm_polarity=[1]  pwm_leading_deadband=[]  pwm_trailing_deadband=[]  initial_pwm_outputs=[0]  final_pwm_outputs=[0]  watchdog_pwm_outputs=[0]  set_pwm_params_at_start=on  set_pwm_params_at_switch_in=off  set_pwm_outputs_at_start=on  set_pwm_outputs_at_switch_in=off  set_pwm_outputs_at_terminate=on  set_pwm_outputs_at_switch_out=off  set_pwm_outputs_on_watchdog=off  other_output_channels=[1000 11000]  initial_other_outputs=[0]  final_other_outputs=[0]  watchdog_other_outputs=[0]  set_other_outputs_at_start=on  set_other_outputs_at_switch_in=off  set_other_outputs_at_terminate=on  set_other_outputs_at_switch_out=off  set_other_outputs_on_watchdog=off
  HIL Read : quarc_library/Data Acquisition/Generic/Immediate I//O/HIL Read  object_name=HIL-1  analog_channels=[4 2]  encoder_channels=[0]  digital_channels=[]  other_channels=[14000 3002 4001]  sample_time=qc_get_step_size  active=on  vector_output=off  data_type_mode=Inherit via back propagation  encoder_data_type=double  digital_data_type=boolean
  HIL Write : quarc_library/Data Acquisition/Generic/Immediate I//O/HIL Write  object_name=HIL-1  analog_channels=[]  pwm_channels=[]  digital_channels=[17:18 25:26 11:16 19:24]  other_channels=[1000 11000]  sample_time=-1  active=off  vector_input=on
  LEDs : Subsystem
  Less Than Threshold1 : Subsystem
  MATLAB Function : MATLAB Function  TreatAsAtomicUnit=on
  Memory : Memory
  Mux : Mux  Inputs=2
  Scope : Scope
  Steering Bias : Bias  Bias=0.05*-1  SaturateOnIntegerOverflow=off
  Unwrap 2^24 : quarc_library/Discontinuities/Inverse Modulus  modulus=16777215  output_derivative=off  output_revolutions=off  max_x=Inf  min_x=-Inf
  basicSpeedEstimation : Subsystem
  basicSpeedEstimation1 : Subsystem
  command saturation : Saturate  UpperLimit=.3  LowerLimit=-0.3
  direction convention : Gain  Gain=+1
  motorCurrent (A) [1] : Outport  VectorParamsAs1DForOutWhenUnconnected=off
  batteryVoltage (V) [1] : Outport  Port=2  VectorParamsAs1DForOutWhenUnconnected=off
  Speed (m/s) : Outport  Port=3  VectorParamsAs1DForOutWhenUnconnected=off
  gyroscopicRates (rad/s) : Outport  Port=4  VectorParamsAs1DForOutWhenUnconnected=off
  Odometer : Outport  Port=5  VectorParamsAs1DForOutWhenUnconnected=off
  wires:
  Demux/2 -> MATLAB Function/1(steering_in), LEDs/2(Steering)
  direction convention/1 -> command saturation/1
  "motorCmd (%, rad) [2]"/1 -> Demux/1
  HIL Read/3 -> Unwrap 2^24/1  "encoder counts"
  Gain/1 -> Steering Bias/1
  HIL Read/1 -> motorCurrent (A) [1]/1  "motor current"
  HIL Read/2 -> batteryVoltage (V) [1]/1  "battery voltage"
  HIL Read/4 -> basicSpeedEstimation/1(motorSpeed (counts/s))
  Unwrap 2^24/1 -> basicSpeedEstimation1/1(motorSpeed (counts/s))
  basicSpeedEstimation1/1(longitudinalCarSpeed (m/s)) -> Odometer/1
  basicSpeedEstimation/1(longitudinalCarSpeed (m/s)) -> [Speed], Speed (m/s)/1
  Demux/1 -> LEDs/1(Throttle), Scope/1, direction convention/1
  HIL Read/5 -> gyroscopicRates (rad/s)/1
  LEDs/1(LEDs) -> HIL Write/1
  Honk/1 -> Audio/1(Honk)
  Arm/1 -> Audio/2(Arm)
  [Speed] -> LEDs/3(Speed)
  Hazard/1 -> LEDs/4(Hazzard)
  HIL Read/6 -> Abs/1
  Abs/1 -> Greater Than Threshold/1(Signal)
  Constant6/1 -> Greater Than Threshold/2(Threshold)
  Constant1/1 -> Greater Than Threshold/3(Duration)
  Greater Than Threshold/1(elapsed) -> Audio/3(put_me_down)
  Volume/1 -> Audio/4(Volume)
  Constant3/1 -> Less Than Threshold1/2(Threshold)
  Constant4/1 -> Less Than Threshold1/3(Duration)
  [Speed] -> Less Than Threshold1/1(Signal)
  MATLAB Function/1(steering_out) -> Gain/1, Memory/1
  Less Than Threshold1/1(elapsed) -> Display/1, MATLAB Function/2(stopped)
  Memory/1 -> MATLAB Function/3(previous_steering)
  Mux/1 -> HIL Write/2
  Steering Bias/1 -> Mux/1
  command saturation/1 -> Mux/2

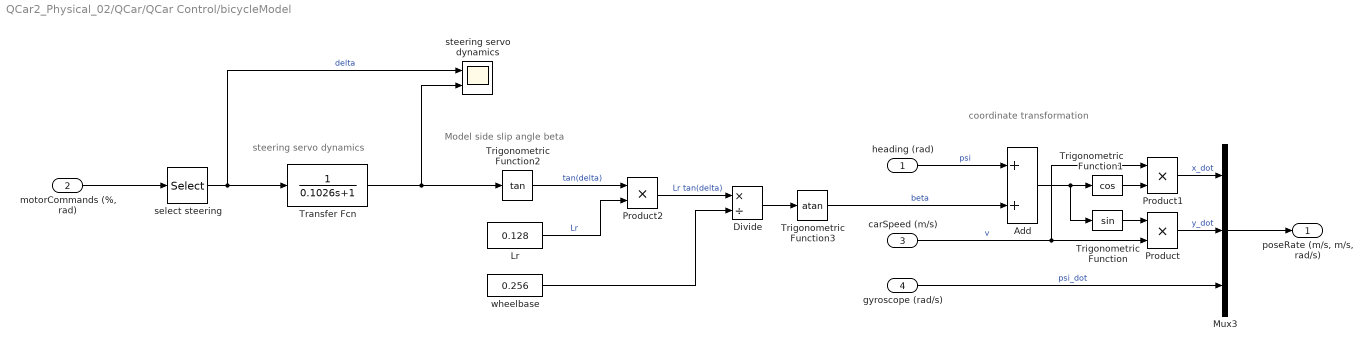
== system QCar2_Physical_02/QCar/QCar Control/bicycleModel ==
  note: coordinate transformation
  note: Model side slip angle beta
  note: steering servo dynamics
  heading (rad) : Inport
  "motorCommands (%, rad)" : Inport  Port=2
  carSpeed (m/s) : Inport  Port=3
  gyroscope (rad/s) : Inport  Port=4
  Add : Sum
  Divide : Product  Inputs=*/
  Lr : Constant  Value=0.128
  Mux3 : Mux  Inputs=3
  Product : Product
  Product1 : Product
  Product2 : Product
  Transfer Fcn : TransferFcn  Denominator=[0.1026 1]
  Trigonometric Function : Trigonometry
  Trigonometric Function1 : Trigonometry  Operator=cos
  Trigonometric Function2 : Trigonometry  Operator=tan
  Trigonometric Function3 : Trigonometry  Operator=atan
  select steering : Selector  InputPortWidth=2  IndexOptions=Index vector (dialog)  Indices=[2]  OutputSizes=1
  steering servo dynamics : Scope  NumInputPorts=2
  wheelbase : Constant  Value=0.256
  "poseRate (m/s, m/s, rad/s)" : Outport  VectorParamsAs1DForOutWhenUnconnected=off
  wires:
  Add/1 -> Trigonometric Function1/1, Trigonometric Function/1
  Trigonometric Function1/1 -> Product1/2
  Product/1 -> Mux3/2  "y_dot"
  select steering/1 -> Transfer Fcn/1, steering servo dynamics/1  "delta"
  carSpeed (m/s)/1 -> Product/2, Product1/1  "v"
  Product1/1 -> Mux3/1  "x_dot"
  Trigonometric Function/1 -> Product/1
  gyroscope (rad/s)/1 -> Mux3/3  "psi_dot"
  heading (rad)/1 -> Add/1  "psi"
  "motorCommands (%, rad)"/1 -> select steering/1
  Mux3/1 -> "poseRate (m/s, m/s, rad/s)"/1
  Transfer Fcn/1 -> Trigonometric Function2/1, steering servo dynamics/2
  Divide/1 -> Trigonometric Function3/1
  wheelbase/1 -> Divide/2
  Product2/1 -> Divide/1  "Lr tan(delta)"
  Trigonometric Function3/1 -> Add/2  "beta"
  Trigonometric Function2/1 -> Product2/1  "tan(delta)"
  Lr/1 -> Product2/2  "Lr"

== system QCar2_Physical_02/QCar/QCar Control/powerConsumptionMonitor ==
  note: Battery percentage calculation
  note: P = VI
  note: Electrical
      | power
      | consumed
  note: Power Monitoring Module:
      |
      | This subsystem monitors power consumption and provides a percentage battery remaining indicator.
      |
      | Inputs:
      | motorCurrent (A) n/a : Motor current being pulled by the main drive motor
      | batteryVoltage (V) {0, 12.6} : Current battery voltage reading
      |
      | Outputs:
      | motorPowerConsumption (W) n/a : Current power in Watts being pulled by the main drive motor
      | batteryLevel (%) {0,1} : Percentage battery level remaining
      |
      | Usage:
      | This is based on a maximum 3S battery voltage of 12.6 V (4.2V per cell) and minimum of 10.5 V (3.5V per cell)
  motorCurrent (A) [1] : Inport
  batteryVoltage (V) [1] : Inport  Port=2
  Divide : Product  Inputs=*/
  Gain : Gain  Gain=100
  Product : Product
  Subtract : Sum  Inputs=+-
  Subtract1 : Sum  Inputs=+-
  max voltage : Constant  Value=12.6
  min voltage : Constant  Value=10.5
  motorPowerConsumption (W) [1] : Outport  VectorParamsAs1DForOutWhenUnconnected=off
  batteryLevel (%) [1] : Outport  Port=2  VectorParamsAs1DForOutWhenUnconnected=off
  wires:
  Divide/1 -> Gain/1
  Subtract1/1 -> Divide/2
  Gain/1 -> batteryLevel (%) [1]/1
  Product/1 -> motorPowerConsumption (W) [1]/1
  min voltage/1 -> Subtract/2, Subtract1/2
  motorCurrent (A) [1]/1 -> Product/1
  max voltage/1 -> Subtract1/1
  Subtract/1 -> Divide/1
  batteryVoltage (V) [1]/1 -> Subtract/1, Product/2

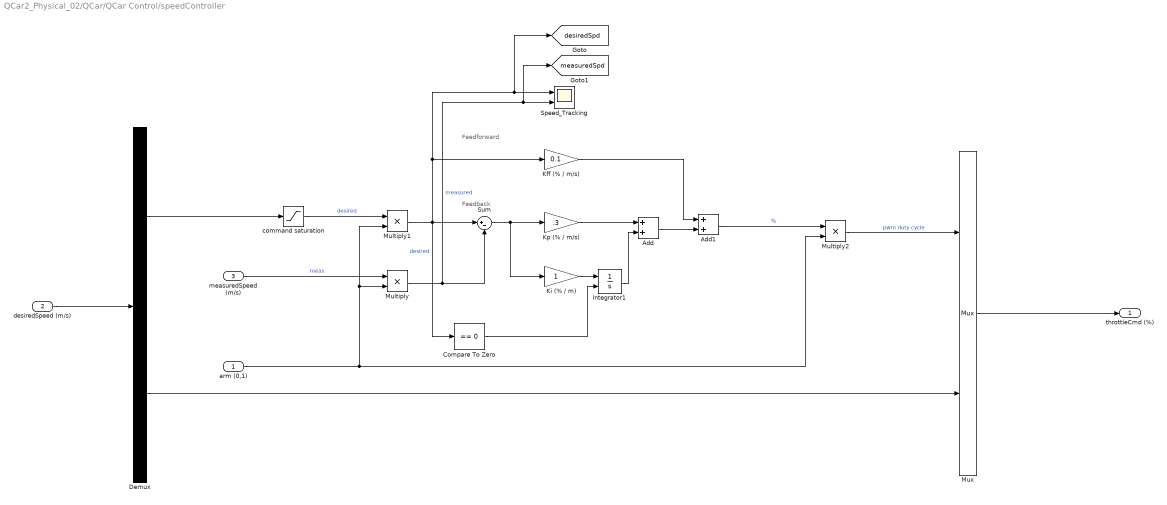
== system QCar2_Physical_02/QCar/QCar Control/speedController ==
  note: Feedforward
  note: Feedback
  arm (0,1) : Inport
  desiredSpeed (m/s) : Inport  Port=2
  measuredSpeed (m/s) : Inport  Port=3
  Add : Sum
  Add1 : Sum
  Compare To Zero : simulink/Logic and Bit Operations/Compare To Zero  relop===  OutDataTypeStr=boolean
  Demux : Demux  Outputs=2
  Integrator1 : Integrator  ExternalReset=either  LimitOutput=on  UpperSaturationLimit=0.4  LowerSaturationLimit=-0.4
  Kff (% / m/s) : Gain  Gain=0.1
  "Ki (% / m) " : Gain
  Kp (% / m/s) : Gain  Gain=.3
  Multiply : Product
  Multiply1 : Product
  Multiply2 : Product
  Mux : Mux  Inputs=2
  Speed_Tracking : Scope  NumInputPorts=2
  Sum : Sum  Inputs=|+-
  command saturation : Saturate  UpperLimit=5  LowerLimit=-5
  throttleCmd (%) : Outport  VectorParamsAs1DForOutWhenUnconnected=off
  tag scope: desiredSpd=global, measuredSpd=global
  wires:
  command saturation/1 -> Multiply1/1  "desired"
  arm (0,1)/1 -> Multiply1/2, Multiply/2, Multiply2/2
  measuredSpeed (m/s)/1 -> Multiply/1  "meas"
  Multiply/1 -> Sum/2, [measuredSpd], Speed_Tracking/2  "measured"
  Add/1 -> Add1/2
  Add1/1 -> Multiply2/1  "%"
  Multiply1/1 -> Compare To Zero/1, Sum/1, Kff (% / m/s)/1, [desiredSpd], Speed_Tracking/1  "desired"
  Integrator1/1 -> Add/2
  Kp (% / m/s)/1 -> Add/1
  Compare To Zero/1 -> Integrator1/2
  Kff (% / m/s)/1 -> Add1/1
  Sum/1 -> "Ki (% / m) "/1, Kp (% / m/s)/1
  "Ki (% / m) "/1 -> Integrator1/1
  Multiply2/1 -> Mux/1  "pwm duty cycle"
  Mux/1 -> throttleCmd (%)/1
  desiredSpeed (m/s)/1 -> Demux/1
  Demux/1 -> command saturation/1
  Demux/2 -> Mux/2

== system QCar2_Physical_02/QCar/QCar Control/turnSpeedHandling ==
  Commands in : Inport
  Cos ^ : Inport  Port=2
  Cos : Trigonometry  Operator=cos
  Demux1 : Demux  Outputs=2
  Mux : Mux  Inputs=2
  Product : Product
  Saturation : Saturate  UpperLimit=1  LowerLimit=.3
  Scope : Scope  NumInputPorts=2
  Scope1 : Scope  NumInputPorts=2
  Square : Math  Operator=pow  SignedPower=on
  Commands : Outport  VectorParamsAs1DForOutWhenUnconnected=off
  wires:
  Cos/1 -> Square/1
  Saturation/1 -> Product/2
  Demux1/1 -> Product/1, Scope/1  "Speed Command"
  Commands in/1 -> Demux1/1
  Cos ^/1 -> Square/2
  Square/1 -> Saturation/1, Scope1/1
  Product/1 -> Mux/1, Scope/2
  Mux/1 -> Commands/1
  Demux1/2 -> Mux/2, Scope1/2, Cos/1
